simulink model "LMI_alocacao_statefeedback"  (Simulink 7.7)
settings: Solver=ode45  StartTime=0.0  StopTime=2000  RelTol=1e-3
values from neighbouring files (symbols this model uses):
  QT =     [FaseMinima.mat]    (also in FaseNaoMinima.mat; FaseNaoMinimaMudandoApenasGama.mat; settup.m = dynamics())
settings Model: Creator=Arthur  LastModifiedBy=Arthur
settings DebuggingCC: UnderspecifiedInitializationDetection=Simplified

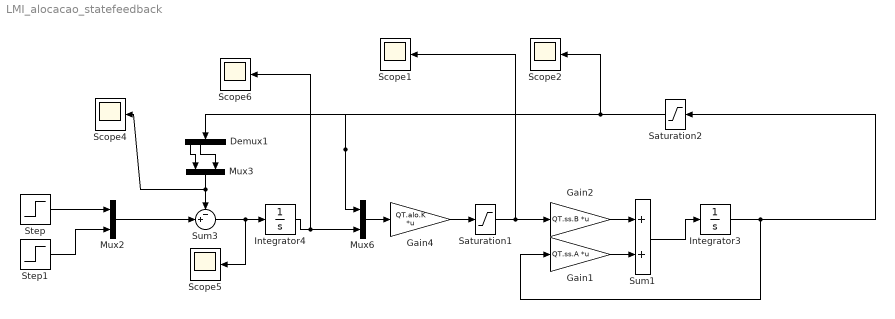
== system LMI_alocacao_statefeedback ==
  Demux1 : Demux
  Gain1 : Gain  Gain=QT.ss.A  Multiplication=Matrix(K*u)
  Gain2 : Gain  Gain=QT.ss.B  Multiplication=Matrix(K*u)
  Gain4 : Gain  Gain=QT.alo.K  Multiplication=Matrix(K*u)
  Integrator3 : Integrator
  Integrator4 : Integrator
  Mux2 : Mux  Inputs=2
  Mux3 : Mux  Inputs=2
  Mux6 : Mux  Inputs=2
  Saturation1 : Saturate  UpperLimit=1.5  LowerLimit=-1.5
  Saturation2 : Saturate  UpperLimit=10  LowerLimit=-10
  Scope{1..2,4..6} (5 alike) : Scope
      Scope1 settings: YMin=-0.75  YMax=2.25  SampleInput=on  SampleTime=1
      Scope2 settings: YMin=-0.75  YMax=2.25  SampleInput=on  SampleTime=1
      Scope4 settings: YMin=-0.75  YMax=2.25  SaveName=ScopeData3  SampleInput=on  SampleTime=1
      Scope5 settings: YMin=-0.75  YMax=2.25  SaveName=ScopeData4  SampleTime=1
      Scope6 settings: YMin=-0.75  YMax=2.25  SaveName=ScopeData5  SampleInput=on  SampleTime=1
  Step : Step  Time=1000  SampleTime=0
  Step1 : Step  Time=500  SampleTime=0
  Sum1 : Sum
  Sum3 : Sum  Inputs=-+|
  wires:
  Step/1 -> Mux2/1
  Step1/1 -> Mux2/2
  Mux2/1 -> Sum3/2
  Gain1/1 -> Sum1/2
  Gain2/1 -> Sum1/1
  Integrator3/1 -> Gain1/1, Saturation2/1
  Sum1/1 -> Integrator3/1
  Gain4/1 -> Saturation1/1
  Mux6/1 -> Gain4/1
  Integrator4/1 -> Mux6/2, Scope6/1
  Sum3/1 -> Integrator4/1, Scope5/1
  Demux1/1 -> Mux3/1
  Demux1/2 -> Mux3/2
  Mux3/1 -> Sum3/1, Scope4/1
  Saturation2/1 -> Mux6/1, Demux1/1, Scope2/1
  Saturation1/1 -> Gain2/1, Scope1/1
